simulink model "untitled"  (R2021a)
settings: Solver=VariableStepAuto  StartTime=0.0  StopTime=10.0  RelTol=1e-3
libraries: sharedtransform x1
settings Model: Creator=Owner  LastModifiedBy=Owner

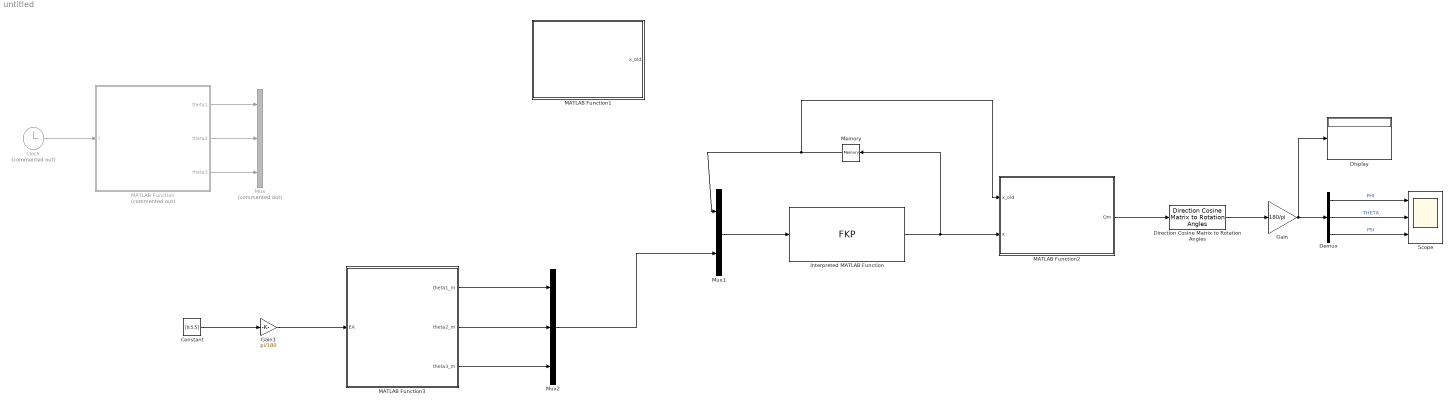
== system untitled ==
  Clock : Clock  Commented=on
  Constant : Constant  Value=[0;5;5]
  Demux : Demux  Outputs=3
  Direction Cosine Matrix to Rotation Angles : sharedtransform/Direction Cosine Matrix to Rotation Angles  rotationOrder=XYZ  aMode=aMode  action=None  tolerance=eps(2)
      settings: SourceProductBaseCode=AE,PW,DR,MT,UV,VE
  Display : Display
  Gain : Gain  Gain=180/pi
  Gain1 : Gain  Gain=pi/180
  Interpreted MATLAB Function : MATLABFcn  MATLABFcn=FKP  OutputDimensions=9  Output1D=off
  MATLAB Function : MATLAB Function  Commented=on  TreatAsAtomicUnit=on
  MATLAB Function1 : MATLAB Function  TreatAsAtomicUnit=on
  MATLAB Function2 : MATLAB Function  TreatAsAtomicUnit=on
  MATLAB Function3 : MATLAB Function  TreatAsAtomicUnit=on
  Memory : Memory
  Mux : Mux  Commented=on  Inputs=3
  Mux1 : Mux  Inputs=2
  Mux2 : Mux  Inputs=3
  Scope : Scope  NumInputPorts=3
  wires:
  Clock/1 -> MATLAB Function/1(t)
  MATLAB Function/3(theta3) -> Mux/3
  MATLAB Function/2(theta2) -> Mux/2
  MATLAB Function/1(theta1) -> Mux/1
  MATLAB Function2/1(Qm) -> Direction Cosine Matrix to Rotation Angles/1
  Direction Cosine Matrix to Rotation Angles/1 -> Gain/1
  Mux1/1 -> Interpreted MATLAB Function/1
  Interpreted MATLAB Function/1 -> Memory/1, MATLAB Function2/2(x)
  MATLAB Function3/1(theta1_m) -> Mux2/1
  MATLAB Function3/2(theta2_m) -> Mux2/2
  MATLAB Function3/3(theta3_m) -> Mux2/3
  Mux2/1 -> Mux1/2
  Gain1/1 -> MATLAB Function3/1(EA)
  Constant/1 -> Gain1/1
  Demux/1 -> Scope/1  "PHI"
  Demux/2 -> Scope/2  "THETA"
  Demux/3 -> Scope/3  "PSI"
  Gain/1 -> Display/1, Demux/1
  Memory/1 -> MATLAB Function2/1(x_old), Mux1/1

== matlab function untitled/MATLAB Function1 ==
  data: x_old output
function x_old = InitialGuess

%% UNIT CONVERTION
dg2rd = pi/180;
rd2dg = 1/dg2rd;
mm2m = 10^(-3);
I2 = eye(2);
I3 = eye(3);
O3 = zeros(3);
I6 = eye(6);
Nm2Nmm = 1e3;

%% GEOMETRIC PARAMETERS
a1s = 65*dg2rd; sa1s = sin(a1s); ca1s = cos(a1s);
a2s = 60*dg2rd; sa2s = sin(a2s); ca2s = cos(a2s);
b1s = 0*dg2rd; sb1s = sin(b1s); cb1s = cos(b1s);
b2s = 110*dg2rd; sb2s = sin(b2s); cb2s = cos(b2s);
ETA = [0;240;120]*dg2rd;
eta1s = 0*dg2rd; se1s = sin(eta1s); ce1s = cos(eta1s);
eta2s = 240*dg2rd; se2s = sin(eta2s); ce2s = cos(eta2s);
eta3s = 120*dg2rd; se3s = sin(eta3s); ce3s = cos(eta3s);
gravity = [0;0;-9.80665];
thetaZ0 = -1.140243740887195*ones(3,1);

%% UNIT VECTORS CONSTANTS

u1v = [sb1s*se1s;sb1s*ce1s;-cb1s];
u2v = [sb1s*se2s;sb1s*ce2s;-cb1s];
u3v = [sb1s*se3s;sb1s*ce3s;-cb1s];
v1v_str = [sb2s*se1s;sb2s*ce1s;cb2s];
v2v_str = [sb2s*se2s;sb2s*ce2s;cb2s];
v3v_str = [sb2s*se3s;sb2s*ce3s;cb2s];

x_old = [v1v_str;v2v_str;v3v_str];


end

== matlab function untitled/MATLAB Function ==
  data: t input; theta1 output; theta2 output; theta3 output
function [theta1,theta2,theta3] = EA_TRAJECTORY(t)


thetaZ0 = -1.140243740887195*ones(3,1);
q1 = -3.195*(pi/180); q2 = 1.856*(pi/180); q3 = 1.599*(pi/180);


theta1 = q1-thetaZ0(1);
theta2 = q2-thetaZ0(2);
theta3 = q3-thetaZ0(3);



end

== matlab function untitled/MATLAB Function2 ==
  data: x_old input; x input; Qm output
function Qm = Convert2DCM(x_old,x)


Vm_new = [x(1:3),x(4:6),x(7:9)];
Vm_OLD = [x_old(1:3),x_old(4:6),x_old(7:9)];

Qm = (Vm_new*Vm_OLD^(-1));



end

== matlab function untitled/MATLAB Function3 ==
  data: EA input; theta1_m output; theta2_m output; theta3_m output
function [theta1_m,theta2_m,theta3_m] = INVERSE_KINEMATIC(EA)

%% UNIT CONVERTION
dg2rd = pi/180;
rd2dg = 1/dg2rd;
mm2m = 10^(-3);
I2 = eye(2);
I3 = eye(3);
O3 = zeros(3);
I6 = eye(6);
Nm2Nmm = 1e3;

%% GEOMETRIC PARAMETERS
a1s = 65*dg2rd; sa1s = sin(a1s); ca1s = cos(a1s);
a2s = 60*dg2rd; sa2s = sin(a2s); ca2s = cos(a2s);
b1s = 0*dg2rd; sb1s = sin(b1s); cb1s = cos(b1s);
b2s = 110*dg2rd; sb2s = sin(b2s); cb2s = cos(b2s);
ETA = [0;240;120]*dg2rd;
eta1s = 0*dg2rd; se1s = sin(eta1s); ce1s = cos(eta1s);
eta2s = 240*dg2rd; se2s = sin(eta2s); ce2s = cos(eta2s);
eta3s = 120*dg2rd; se3s = sin(eta3s); ce3s = cos(eta3s);
gravity = [0;0;-9.80665];
thetaZ0 = -1.140243740887195*ones(3,1);

%% UNIT VECTORS CONSTANTS

u1v = [sb1s*se1s;sb1s*ce1s;-cb1s];
u2v = [sb1s*se2s;sb1s*ce2s;-cb1s];
u3v = [sb1s*se3s;sb1s*ce3s;-cb1s];
v1v_str = [sb2s*se1s;sb2s*ce1s;cb2s];
v2v_str = [sb2s*se2s;sb2s*ce2s;cb2s];
v3v_str = [sb2s*se3s;sb2s*ce3s;cb2s];

RX= [1 0 0; 0 cos(EA(1)) -sin(EA(1)); 0 sin(EA(1)) cos(EA(1));];
RY=[cos(EA(2)) 0 sin(EA(2)); 0 1 0; -sin(EA(2)) 0 cos(EA(2));];
RZ=[cos(EA(3)) -sin(EA(3)) 0; sin(EA(3)) cos(EA(3)) 0; 0 0 1;];


Qm = RZ*RY*RX;
v1v = Qm*v1v_str;
v2v = Qm*v2v_str;
v3v = Qm*v3v_str;
%% ---LEG1----
A1_1 = sin(a1s-b1s)*(se1s*v1v(1)+ce1s*v1v(2))+cos(a1s-b1s)*v1v(3)+ca2s;
B1_1 = sa1s*(ce1s*v1v(1)-se1s*v1v(2));
C1_1 = -sin(a1s+b1s)*(se1s*v1v(1)+ce1s*v1v(2))+cos(a1s+b1s)*(v1v(3))+ca2s;
D1_1 = B1_1^2-A1_1*C1_1;
T11_1 = (-B1_1+sqrt(D1_1))/A1_1;
T12_1 = (-B1_1-sqrt(D1_1))/A1_1;
theta1_p = 2*atan(T11_1);
theta1_m = 2*atan(T12_1);
theta1 = theta1_m;

%% ---LEG2----
A2_1 = sin(a1s-b1s)*(se2s*v2v(1)+ce2s*v2v(2))+cos(a1s-b1s)*v2v(3)+ca2s;
B2_1 = sa1s*(ce2s*v2v(1)-se2s*v2v(2));
C2_1 = -sin(a1s+b1s)*(se2s*v2v(1)+ce2s*v2v(2))+cos(a1s+b1s)*(v2v(3))+ca2s;
D2_1 = B2_1^2-A2_1*C2_1;
T21_1 = (-B2_1+sqrt(D2_1))/A2_1;
T22_1 = (-B2_1-sqrt(D2_1))/A2_1;
theta2_p = 2*atan(T21_1);
theta2_m = 2*atan(T22_1);
theta2 = theta2_m;


%% ---LEG3----
A3_1 = sin(a1s-b1s)*(se3s*v3v(1)+ce3s*v3v(2))+cos(a1s-b1s)*v3v(3)+ca2s;
B3_1 = sa1s*(ce3s*v3v(1)-se3s*v3v(2));
C3_1 = -sin(a1s+b1s)*(se3s*v3v(1)+ce3s*v3v(2))+cos(a1s+b1s)*(v3v(3))+ca2s;
D3_1= B3_1^2-A3_1*C3_1;
T31_1 = (-B3_1+sqrt(D3_1))/A3_1;
T32_1 = (-B3_1-sqrt(D3_1))/A3_1;
theta3_p = 2*atan(T31_1);
theta3_m = 2*atan(T32_1);
theta3 = theta3_m;


end
